simulink model "sedemo_fifo_architectural"  (Simulink 7.5)
settings: Solver=VariableStepDiscrete  StartTime=0.0  StopTime=10  MaxStep=inf  RelTol=1e-3
undefined symbols (not defined in the file or in its folder): des_subsystemblock, des_subsysteminport, des_subsystemoutport, des_subsystemsupportblock
libraries: simeventstranslate1 x16, simeventssink1 x5, simulink x2, simeventsgenerators1 x2, simeventsqueue1 x2, simeventsattributes2 x2, simeventsgates1 x2, simeventsserver1 x2, simeventssignalmanage1 x1, simeventsinfo x1, simeventsrouting1 x1
(part 1 of 2)
settings Model: Creator=The MathWorks Inc.  ExtModeAutoUpdateStatusClock=off
settings DataIOCC: SaveOutput=off  SaveTime=off
settings OptimizationCC: InitFltsAndDblsToZero=on  EfficientMapNaN2IntZero=off
settings DebuggingCC: ReadBeforeWriteMsg=DisableAll  WriteAfterWriteMsg=DisableAll  WriteAfterReadMsg=DisableAll  AlgebraicLoopMsg=error  SolverPrmCheckMsg=none  StrictBusMsg=Warning
settings SimEventsCC: propDiagAttribOutput=1  propDiagFcnCallOutput=1  propDiagStatOutput=0

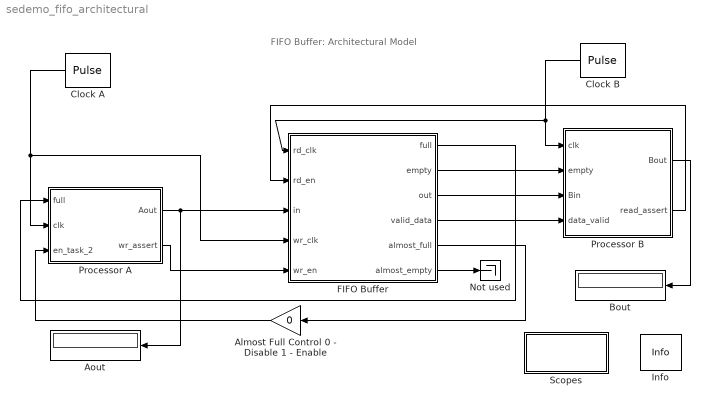
== system sedemo_fifo_architectural ==
  note: FIFO Buffer: Architectural Model
  Almost Full Control 0 - Disable 1 - Enable : Gain  Gain=0  ParameterDataType=sfix(16)  ParameterScaling=2^0  OutDataType=sfix(16)  OutScaling=2^0
  Aout : Display
  Bout : Display
  Clock A : DiscretePulseGenerator  PulseType=Time based  Amplitude=1  Period=0.005  PulseWidth=50  PhaseDelay=0  SampleTime=1
      settings: AttributesFormatString=Period = %<Period>
  Clock B : DiscretePulseGenerator  PulseType=Time based  Amplitude=1  Period=0.0065  PulseWidth=50  PhaseDelay=0  SampleTime=1
      settings: AttributesFormatString=Period = %<Period>
  FIFO Buffer : Subsystem  mask(Variable Capacity, Variable Space per Entity Buffer){thresholdLow=40, thresholdHigh=240, FQcapacity=256}
      mask prompts: thresholdLow "Low Water Level"; thresholdHigh "High Water Level"; FQcapacity "Capacity"
      mask help: Variable capacity queue that allows entities to occupy a variable amount of space per entitiy. The amount of space from an entity is specified from the attribute named in the dialog.
  Info : simeventsinfo/Info  SystemSampleTime=-1
  Not used : Terminator
  Processor A : Subsystem
  Processor B : Subsystem
  Scopes : Subsystem
      settings: RequestExecContextInheritance=on
      mask Display: disp('Scopes');
  wires:
  Clock A/1 -> Processor A/2(clk), FIFO Buffer/4(wr_clk)
  Clock B/1 -> FIFO Buffer/1(rd_clk), Processor B/1(clk)
  FIFO Buffer/3(out) -> Processor B/3(Bin)
  Processor A/1(Aout) -> Aout/1, FIFO Buffer/3(in)
  Processor B/1(Bout) -> Bout/1
  Processor B/2(read_assert) -> FIFO Buffer/2(rd_en)
  Processor A/2(wr_assert) -> FIFO Buffer/5(wr_en)
  FIFO Buffer/1(full) -> Processor A/1(full)
  FIFO Buffer/2(empty) -> Processor B/2(empty)
  FIFO Buffer/4(valid_data) -> Processor B/4(data_valid)
  FIFO Buffer/5(almost_full) -> Almost Full Control 0 - Disable 1 - Enable/1
  FIFO Buffer/6(almost_empty) -> Not used/1
  Almost Full Control 0 - Disable 1 - Enable/1 -> Processor A/3(en_task_2)

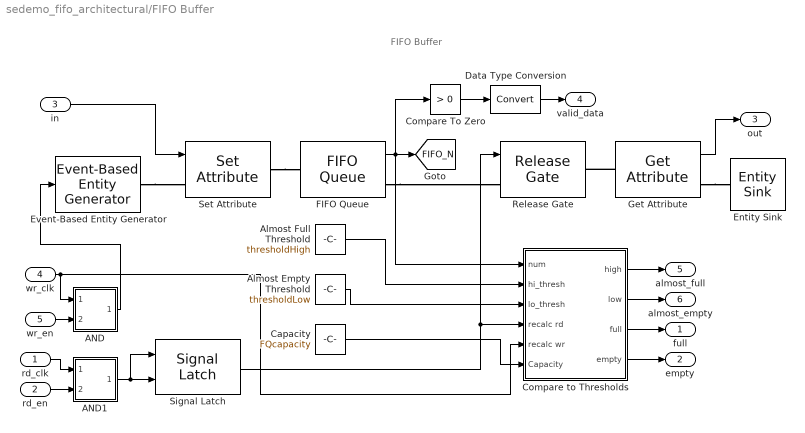
== system sedemo_fifo_architectural/FIFO Buffer ==
  note: FIFO Buffer
  rd_clk : Inport
  rd_en : Inport  Port=2
  in : Inport  Port=3
  wr_clk : Inport  Port=4
  wr_en : Inport  Port=5
  AND : Subsystem  LoadFcn=des_subsystemblock(gcb, 'load');  InitFcn=des_subsystemblock(gcb, 'init');  StartFcn=des_subsystemblock(gcb, 'start');  StopFcn=des_subsystemblock(gcb, 'stop');
      settings: CopyFcn=des_subsystemblock(gcb, 'copy');  DeleteFcn=des_subsystemblock(gcb, 'delete');  UndoDeleteFcn=des_subsystemblock(gcb, 'undodelete');  ModelCloseFcn=des_subsystemblock(gcb, 'modelclose');  PreSaveFcn=des_subsystemblock(gcb, 'presave');  NameChangeFcn=des_subsystemblock(gcb, 'namechange');  OpenFcn=des_subsystemblock(gcb, 'open');  ParentCloseFcn=des_subsystemblock(gcb, 'parentclose');  ErrorFcn=des_subsystemerror
      mask Type: Discrete Event Subsystem
      mask Help: helpview(simeventsbhelp);
  AND1 : Subsystem  LoadFcn=des_subsystemblock(gcb, 'load');  InitFcn=des_subsystemblock(gcb, 'init');  StartFcn=des_subsystemblock(gcb, 'start');  StopFcn=des_subsystemblock(gcb, 'stop');
      settings: CopyFcn=des_subsystemblock(gcb, 'copy');  DeleteFcn=des_subsystemblock(gcb, 'delete');  UndoDeleteFcn=des_subsystemblock(gcb, 'undodelete');  ModelCloseFcn=des_subsystemblock(gcb, 'modelclose');  PreSaveFcn=des_subsystemblock(gcb, 'presave');  NameChangeFcn=des_subsystemblock(gcb, 'namechange');  OpenFcn=des_subsystemblock(gcb, 'open');  ParentCloseFcn=des_subsystemblock(gcb, 'parentclose');  ErrorFcn=des_subsystemerror
      mask Type: Discrete Event Subsystem
      mask Help: helpview(simeventsbhelp);
  Almost Empty Threshold : Constant  Value=thresholdLow  OutDataType=sfix(16)  OutScaling=2^0
  Almost Full Threshold : Constant  Value=thresholdHigh  OutDataType=sfix(16)  OutScaling=2^0
  Capacity : Constant  Value=FQcapacity  OutDataType=sfix(16)  OutScaling=2^0
  Compare To Zero : simulink/Logic and Bit Operations/Compare To Zero  SystemSampleTime=-1  relop=>  LogicOutDataTypeMode=uint8  ZeroCross=off
  Compare to Thresholds : Subsystem  LoadFcn=des_subsystemblock(gcb, 'load');  InitFcn=des_subsystemblock(gcb, 'init');  StartFcn=des_subsystemblock(gcb, 'start');  StopFcn=des_subsystemblock(gcb, 'stop');
      settings: CopyFcn=des_subsystemblock(gcb, 'copy');  DeleteFcn=des_subsystemblock(gcb, 'delete');  UndoDeleteFcn=des_subsystemblock(gcb, 'undodelete');  ModelCloseFcn=des_subsystemblock(gcb, 'modelclose');  PreSaveFcn=des_subsystemblock(gcb, 'presave');  NameChangeFcn=des_subsystemblock(gcb, 'namechange');  OpenFcn=des_subsystemblock(gcb, 'open');  ParentCloseFcn=des_subsystemblock(gcb, 'parentclose');  ErrorFcn=des_subsystemerror
      mask Type: Discrete Event Subsystem
      mask Help: helpview(simeventsbhelp);
  Data Type Conversion : DataTypeConversion  OutDataType=sfix(16)  OutScaling=2^0
  Entity Sink : simeventssink1/Entity Sink  Priority=1  SystemSampleTime=-1  AvailableForArrivals=on  StatNumberArrived=Off
  Event-Based Entity Generator : simeventsgenerators1/Entity Generators/Event-Based Entity Generator  Priority=1  DialogController=des_ddg_create  DialogControllerArgs=DataTag40  SystemSampleTime=-1  GenerateEntitiesUpon=Trigger from port tr  SignalEdgeType=Rising  SpecifyEventPriority=off  PriorityEntityGeneration=300  GenerateEntityAtSimulationStart=off  AllowBlocking=off  ResponseDuringBlockage=Delay first pending entity  EntityType=Blank  StatNumberDeparted=Off  StatPendingEntity=Off  StatAverageIntergenerationTime=Off
  FIFO Queue : simeventsqueue1/FIFO Queue  Priority=1  SystemSampleTime=-1  Capacity=inf  EnableTOPort=off  StatNumberDeparted=Off  StatNumberInBlock=On  StatPendingEntity=Off  StatAverageWait=Off  StatAverageQueueLength=Off  StatNumberTimedout=Off
  Get Attribute : simeventsattributes2/Get Attribute  Priority=1  DialogController=des_ddg_create  DialogControllerArgs=DataTag43  SystemSampleTime=-1  AttributeName=Attribute1  AttributeMissing=Error  AttributeDefaultValue=1  AttributeSendTiming=After entity departure  AttributeTreatAsVector=1  StatNumberDeparted=Off  EvaluatedDefaultAttributeValue={[]}
  Release Gate : simeventsgates1/Release Gate  Priority=1  SystemSampleTime=-1  OpenGateUpon=Trigger from port tr  SignalEdgeOption=Rising  SpecifyEventPriority=off  PriorityGateRelease=2200  StatNumberDeparted=Off
  Set Attribute : simeventsattributes2/Set Attribute  Priority=1  DialogController=des_ddg_create  DialogControllerArgs=DataTag46  SystemSampleTime=-1  AttributeFrom=Signal port|Dialog  AttributeName=Attribute1|space  AttributeTreatAsVector=1|1  AttributeValue=1|1  AttributeCreate=on  StatNumberDeparted=Off  EvaluatedAttributeValue={[];1}
  Signal Latch : simeventssignalmanage1/Signal Latch  SystemSampleTime=-1  InitialMemoryValue=0  WriteMemoryUpon=Sample time hit from port wts  MemoryWriteEdgeOption=Rising  SpecifyWriteEventPriority=on  PriorityMemoryWrite=7100  ReadMemoryUpon=Write to memory event  MemoryReadEdgeOption=Falling  SpecifyReadEventPriority=on  PriorityMemoryRead=7000  ReportMemoryState=off  ReportMemoryUponWrite=off  ReportMemoryUponRead=on
  full : Outport  OutDataType=sfix(16)  OutScaling=2^0
  empty : Outport  Port=2  OutDataType=sfix(16)  OutScaling=2^0
  out : Outport  Port=3
  valid_data : Outport  Port=4  OutDataType=sfix(16)  OutScaling=2^0
  almost_full : Outport  Port=5  OutDataType=sfix(16)  OutScaling=2^0
  almost_empty : Outport  Port=6  OutDataType=sfix(16)  OutScaling=2^0
  tag scope: FIFO_N=global
  wires:
  Almost Full Threshold/1 -> Compare to Thresholds/2(hi_thresh)
  FIFO Queue/1 -> Compare to Thresholds/1(num), [FIFO_N], Compare To Zero/1
  Compare To Zero/1 -> Data Type Conversion/1
  Data Type Conversion/1 -> valid_data/1
  Almost Empty Threshold/1 -> Compare to Thresholds/3(lo_thresh)
  wr_clk/1 -> Compare to Thresholds/5(recalc wr), AND/1(Din)
  Signal Latch/1 -> Compare to Thresholds/4(recalc rd), Release Gate/1
  rd_clk/1 -> AND1/1(Din)
  rd_en/1 -> AND1/2(Din1)
  AND1/1(Dout) -> Signal Latch/2, Signal Latch/1
  wr_en/1 -> AND/2(Din1)
  in/1 -> Set Attribute/1
  Get Attribute/1 -> out/1
  AND/1(Dout) -> Event-Based Entity Generator/1
  Capacity/1 -> Compare to Thresholds/6(Capacity)
  Compare to Thresholds/1(high) -> almost_full/1
  Compare to Thresholds/2(low) -> almost_empty/1
  Compare to Thresholds/3(full) -> full/1
  Compare to Thresholds/4(empty) -> empty/1
  connections:
  Set Attribute/RConn1 -- FIFO Queue/LConn1
  Get Attribute/LConn1 -- Release Gate/RConn1
  FIFO Queue/RConn1 -- Release Gate/LConn1
  Event-Based Entity Generator/RConn1 -- Set Attribute/LConn1
  Get Attribute/RConn1 -- Entity Sink/LConn1

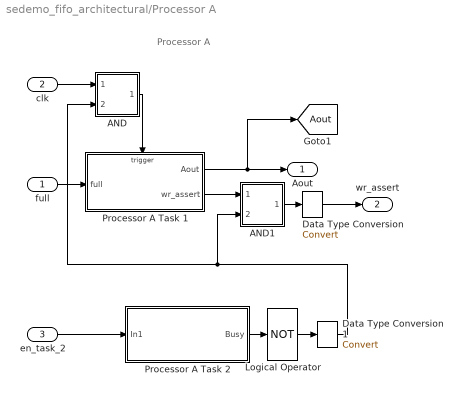
== system sedemo_fifo_architectural/Processor A ==
  note: Processor A
  full : Inport
  clk : Inport  Port=2
  en_task_2 : Inport  Port=3
  AND : Subsystem  LoadFcn=des_subsystemblock(gcb, 'load');  InitFcn=des_subsystemblock(gcb, 'init');  StartFcn=des_subsystemblock(gcb, 'start');  StopFcn=des_subsystemblock(gcb, 'stop');
      settings: CopyFcn=des_subsystemblock(gcb, 'copy');  DeleteFcn=des_subsystemblock(gcb, 'delete');  UndoDeleteFcn=des_subsystemblock(gcb, 'undodelete');  ModelCloseFcn=des_subsystemblock(gcb, 'modelclose');  PreSaveFcn=des_subsystemblock(gcb, 'presave');  NameChangeFcn=des_subsystemblock(gcb, 'namechange');  OpenFcn=des_subsystemblock(gcb, 'open');  ParentCloseFcn=des_subsystemblock(gcb, 'parentclose');  ErrorFcn=des_subsystemerror
      mask Type: Discrete Event Subsystem
      mask Help: helpview(simeventsbhelp);
  AND1 : Subsystem  LoadFcn=des_subsystemblock(gcb, 'load');  InitFcn=des_subsystemblock(gcb, 'init');  StartFcn=des_subsystemblock(gcb, 'start');  StopFcn=des_subsystemblock(gcb, 'stop');
      settings: CopyFcn=des_subsystemblock(gcb, 'copy');  DeleteFcn=des_subsystemblock(gcb, 'delete');  UndoDeleteFcn=des_subsystemblock(gcb, 'undodelete');  ModelCloseFcn=des_subsystemblock(gcb, 'modelclose');  PreSaveFcn=des_subsystemblock(gcb, 'presave');  NameChangeFcn=des_subsystemblock(gcb, 'namechange');  OpenFcn=des_subsystemblock(gcb, 'open');  ParentCloseFcn=des_subsystemblock(gcb, 'parentclose');  ErrorFcn=des_subsystemerror
      mask Type: Discrete Event Subsystem
      mask Help: helpview(simeventsbhelp);
  Data Type Conversion : DataTypeConversion  OutDataType=sfix(16)  OutScaling=2^0
  Data Type Conversion1 : DataTypeConversion  OutDataType=sfix(16)  OutScaling=2^0
  Logical Operator : Logic  Operator=NOT  AllPortsSameDT=off  OutDataTypeMode=boolean  OutDataTypeStr=boolean
  Processor A Task 1 : Subsystem  TreatAsAtomicUnit=on
      settings: PropExecContextOutsideSubsystem=on
  Processor A Task 2 : Subsystem
  Aout : Outport
  wr_assert : Outport  Port=2
  tag scope: Aout=global
  wires:
  Processor A Task 1/1(Aout) -> Aout/1, [Aout]
  full/1 -> Processor A Task 1/1(full)
  en_task_2/1 -> Processor A Task 2/1(In1)
  Processor A Task 2/1(Busy) -> Logical Operator/1
  AND/1(Dout) -> Processor A Task 1/Trigger
  clk/1 -> AND/1(Din)
  AND1/1(Dout) -> Data Type Conversion/1
  Processor A Task 1/2(wr_assert) -> AND1/1(Din)
  Data Type Conversion/1 -> wr_assert/1
  Logical Operator/1 -> Data Type Conversion1/1
  Data Type Conversion1/1 -> AND/2(Din1), AND1/2(Din1)

== system sedemo_fifo_architectural/Processor B ==
  note: Processor B
  clk : Inport
  empty : Inport  Port=2
  Bin : Inport  Port=3
  data_valid : Inport  Port=4
  Not used : Terminator
  Processor B Task : Subsystem  TreatAsAtomicUnit=on
      settings: PropExecContextOutsideSubsystem=on
  Bout : Outport
  read_assert : Outport  Port=2
  tag scope: Bout=global
  wires:
  Bin/1 -> Processor B Task/1(Bin)
  Processor B Task/1(Cout) -> Bout/1, [Bout]
  data_valid/1 -> Not used/1
  empty/1 -> Processor B Task/2(empty)
  Processor B Task/2(read_assert) -> read_assert/1
  clk/1 -> Processor B Task/Trigger

== system sedemo_fifo_architectural/Scopes ==
  Buffer Size : simeventssink1/Signal Scope  Priority=1  SystemSampleTime=-1  PlotType=Stair  InputType=Signal  NumInputs=1  AttributeNameY=Count  XInputOptionSignal=Event time  XInputOptionEntity=Event time  AttributeNameX=Count  EnableEntityOutport=on  XMin=-0.0999478213651573  XMax=10.0947299578809  XLimitExceededOption=Stretch axis limits  YLimitExceededOption=Stretch axis limits  AxisGrid=on  AxisLegend=off  LineDisables=""  LineColors=b  LineStyles=-  LineMarkers=.  OpenScopeAtSimStart=on  Title=Number in Buffer  YLabel=#n  XLabel=Time  FigurePosition=[51 228 231 131]  AxisZoom=off  DataStoreOption=Limited  DataPointsLimit=10000  StatNumberArrived=Off  ShowCountPlotted=off  ShowToolbar=off
      settings: YMin=-2.05  YMax=3.05
  Discrete Event Subsystem Difference : Subsystem  LoadFcn=des_subsystemblock(gcb, 'load');  InitFcn=des_subsystemblock(gcb, 'init');  StartFcn=des_subsystemblock(gcb, 'start');  StopFcn=des_subsystemblock(gcb, 'stop');
      settings: CopyFcn=des_subsystemblock(gcb, 'copy');  DeleteFcn=des_subsystemblock(gcb, 'delete');  UndoDeleteFcn=des_subsystemblock(gcb, 'undodelete');  ModelCloseFcn=des_subsystemblock(gcb, 'modelclose');  PreSaveFcn=des_subsystemblock(gcb, 'presave');  NameChangeFcn=des_subsystemblock(gcb, 'namechange');  OpenFcn=des_subsystemblock(gcb, 'open');  ParentCloseFcn=des_subsystemblock(gcb, 'parentclose');  ErrorFcn=des_subsystemerror
      mask Type: Discrete Event Subsystem
      mask Help: helpview(simeventsbhelp);
  Value of 'A' : simeventssink1/Signal Scope  Priority=1  SystemSampleTime=-1  PlotType=Stair  InputType=Signal  NumInputs=1  AttributeNameY=Count  XInputOptionSignal=Event time  XInputOptionEntity=Event time  AttributeNameX=Count  EnableEntityOutport=on  XMin=-0.0999478213651573  XMax=10.0947299578809  XLimitExceededOption=Stretch axis limits  YLimitExceededOption=Stretch axis limits  AxisGrid=on  AxisLegend=off  LineDisables=""  LineColors=b  LineStyles=-  LineMarkers=.  OpenScopeAtSimStart=on  Title=Value of 'A'  YLabel=""  XLabel=Time  FigurePosition=[294 227 232 134]  AxisZoom=off  DataStoreOption=Limited  DataPointsLimit=10000  StatNumberArrived=Off  ShowCountPlotted=off  ShowToolbar=off
      settings: YMin=-2.05  YMax=3.05
  Value of 'A' - 'B' : simeventssink1/Signal Scope  Priority=1  SystemSampleTime=-1  PlotType=Stair  InputType=Signal  NumInputs=1  AttributeNameY=Count  XInputOptionSignal=Event time  XInputOptionEntity=Event time  AttributeNameX=Count  EnableEntityOutport=on  XMin=-0.0999478213651573  XMax=10.0947299578809  XLimitExceededOption=Stretch axis limits  YLimitExceededOption=Stretch axis limits  AxisGrid=on  AxisLegend=off  LineDisables=""  LineColors=b  LineStyles=-  LineMarkers=.  OpenScopeAtSimStart=on  Title=Value of 'A' - 'B'  YLabel='A' - 'B'  XLabel=Time  FigurePosition=[50 65 231 135]  AxisZoom=off  DataStoreOption=Limited  DataPointsLimit=10000  StatNumberArrived=Off  ShowCountPlotted=off  ShowToolbar=off
      settings: YMin=-2.05  YMax=3.05
  Value of 'B' : simeventssink1/Signal Scope  Priority=1  SystemSampleTime=-1  PlotType=Stair  InputType=Signal  NumInputs=1  AttributeNameY=Count  XInputOptionSignal=Event time  XInputOptionEntity=Event time  AttributeNameX=Count  EnableEntityOutport=on  XMin=-0.0999478213651573  XMax=10.0947299578809  XLimitExceededOption=Stretch axis limits  YLimitExceededOption=Stretch axis limits  AxisGrid=on  AxisLegend=off  LineDisables=""  LineColors=b  LineStyles=-  LineMarkers=.  OpenScopeAtSimStart=on  Title=Value of 'B'  YLabel=""  XLabel=Time  FigurePosition=[294 66 230 136]  AxisZoom=off  DataStoreOption=Limited  DataPointsLimit=10000  StatNumberArrived=Off  ShowCountPlotted=off  ShowToolbar=off
      settings: YMin=-2.05  YMax=3.05
  wires:
  Discrete Event Subsystem Difference/1(Dout) -> Value of 'A' - 'B'/1
  [Aout] -> Discrete Event Subsystem Difference/1(Din), Value of 'A'/1
  [Bout] -> Discrete Event Subsystem Difference/2(Din1), Value of 'B'/1
  [FIFO_N] -> Buffer Size/1

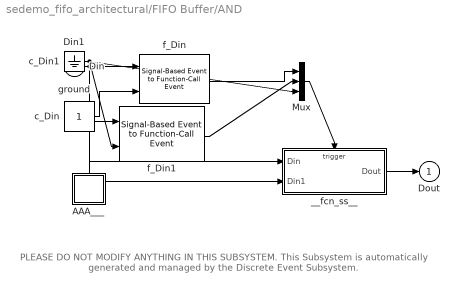
== system sedemo_fifo_architectural/FIFO Buffer/AND ==
  note: PLEASE DO NOT MODIFY ANYTHING IN THIS SUBSYSTEM.
      | This Subsystem is automatically generated and
      | managed by the Discrete Event Subsystem.
  Din : Inport  DataType=double  OutDataType=sfix(16)  OutScaling=2^0  OutDataTypeStr=double
  Din1 : Inport  Port=2  DataType=double  OutDataTypeStr=double
  AAA___ : Subsystem  LoadFcn=des_subsystemsupportblock(gcb, 'load');  InitFcn=des_subsystemsupportblock(gcb, 'init');  StartFcn=des_subsystemsupportblock(gcb, 'start');  StopFcn=des_subsystemsupportblock(gcb, 'stop');
      settings: CopyFcn=des_subsystemsupportblock(gcb, 'copy');  DeleteFcn=des_subsystemsupportblock(gcb, 'delete');  UndoDeleteFcn=des_subsystemsupportblock(gcb, 'undodelete');  ModelCloseFcn=des_subsystemsupportblock(gcb, 'modelclose');  PreSaveFcn=des_subsystemsupportblock(gcb, 'presave');  NameChangeFcn=des_subsystemsupportblock(gcb, 'namechange');  OpenFcn=des_subsystemsupportblock(gcb, 'open');  ParentCloseFcn=des_subsystemsupportblock(gcb, 'parentclose');
  Mux : Mux  Inputs=3
  __fcn_ss__ : Subsystem  TreatAsAtomicUnit=on
      settings: PropExecContextOutsideSubsystem=on
  c_Din : Constant  OutDataType=sfix(16)  OutScaling=2^0
  c_Din1 : Constant
  f_Din : simeventstranslate1/Signal-Based Event to Function-Call Event  Priority=1  SystemSampleTime=-1  GenerateFunctionCallUpon=Sample time hit from port ts  SignalEdgeOption=Rising  EnableE1Port=on  EnableF2Port=off  EnableE2Port=off  SpecifyEventPriority=off  PriorityFunctionCall=20  FunctionCallDelayFrom=Dialog  DelayFunctionCall=0  StatNumberF1Calls=Off  StatNumberF2Calls=Off  MaskBlockType=DESS_EVENT_PORT
  f_Din1 : simeventstranslate1/Signal-Based Event to Function-Call Event  Priority=1  SystemSampleTime=-1  GenerateFunctionCallUpon=Sample time hit from port ts  SignalEdgeOption=Rising  EnableE1Port=on  EnableF2Port=off  EnableE2Port=off  SpecifyEventPriority=off  PriorityFunctionCall=20  FunctionCallDelayFrom=Dialog  DelayFunctionCall=0  StatNumberF1Calls=Off  StatNumberF2Calls=Off  MaskBlockType=DESS_EVENT_PORT
  ground : Ground
  Dout : Outport  OutDataType=sfix(16)  OutScaling=2^0
  wires:
  __fcn_ss__/1(Dout) -> Dout/1
  f_Din/1 -> Mux/1
  c_Din/1 -> f_Din/2
  Mux/1 -> __fcn_ss__/Trigger
  f_Din1/1 -> Mux/2
  c_Din1/1 -> f_Din1/2
  ground/1 -> Mux/3
  Din/1 -> f_Din/1, __fcn_ss__/1(Din)
  Din1/1 -> f_Din1/1, __fcn_ss__/2(Din1)

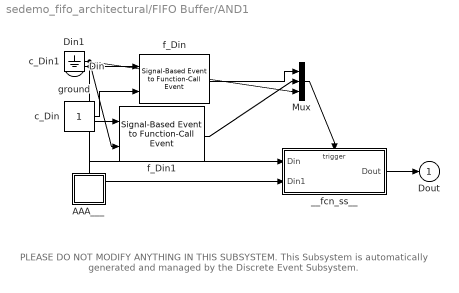
== system sedemo_fifo_architectural/FIFO Buffer/AND1 ==
  note: PLEASE DO NOT MODIFY ANYTHING IN THIS SUBSYSTEM.
      | This Subsystem is automatically generated and
      | managed by the Discrete Event Subsystem.
  Din : Inport  DataType=double  OutDataType=sfix(16)  OutScaling=2^0  OutDataTypeStr=double
  Din1 : Inport  Port=2  DataType=double  OutDataTypeStr=double
  AAA___ : Subsystem  LoadFcn=des_subsystemsupportblock(gcb, 'load');  InitFcn=des_subsystemsupportblock(gcb, 'init');  StartFcn=des_subsystemsupportblock(gcb, 'start');  StopFcn=des_subsystemsupportblock(gcb, 'stop');
      settings: CopyFcn=des_subsystemsupportblock(gcb, 'copy');  DeleteFcn=des_subsystemsupportblock(gcb, 'delete');  UndoDeleteFcn=des_subsystemsupportblock(gcb, 'undodelete');  ModelCloseFcn=des_subsystemsupportblock(gcb, 'modelclose');  PreSaveFcn=des_subsystemsupportblock(gcb, 'presave');  NameChangeFcn=des_subsystemsupportblock(gcb, 'namechange');  OpenFcn=des_subsystemsupportblock(gcb, 'open');  ParentCloseFcn=des_subsystemsupportblock(gcb, 'parentclose');
  Mux : Mux  Inputs=3
  __fcn_ss__ : Subsystem  TreatAsAtomicUnit=on
      settings: PropExecContextOutsideSubsystem=on
  c_Din : Constant  OutDataType=sfix(16)  OutScaling=2^0
  c_Din1 : Constant
  f_Din : simeventstranslate1/Signal-Based Event to Function-Call Event  Priority=1  SystemSampleTime=-1  GenerateFunctionCallUpon=Sample time hit from port ts  SignalEdgeOption=Rising  EnableE1Port=on  EnableF2Port=off  EnableE2Port=off  SpecifyEventPriority=off  PriorityFunctionCall=20  FunctionCallDelayFrom=Dialog  DelayFunctionCall=0  StatNumberF1Calls=Off  StatNumberF2Calls=Off  MaskBlockType=DESS_EVENT_PORT
  f_Din1 : simeventstranslate1/Signal-Based Event to Function-Call Event  Priority=1  SystemSampleTime=-1  GenerateFunctionCallUpon=Sample time hit from port ts  SignalEdgeOption=Rising  EnableE1Port=on  EnableF2Port=off  EnableE2Port=off  SpecifyEventPriority=off  PriorityFunctionCall=20  FunctionCallDelayFrom=Dialog  DelayFunctionCall=0  StatNumberF1Calls=Off  StatNumberF2Calls=Off  MaskBlockType=DESS_EVENT_PORT
  ground : Ground
  Dout : Outport  OutDataType=sfix(16)  OutScaling=2^0
  wires:
  __fcn_ss__/1(Dout) -> Dout/1
  f_Din/1 -> Mux/1
  c_Din/1 -> f_Din/2
  Mux/1 -> __fcn_ss__/Trigger
  f_Din1/1 -> Mux/2
  c_Din1/1 -> f_Din1/2
  ground/1 -> Mux/3
  Din/1 -> f_Din/1, __fcn_ss__/1(Din)
  Din1/1 -> f_Din1/1, __fcn_ss__/2(Din1)

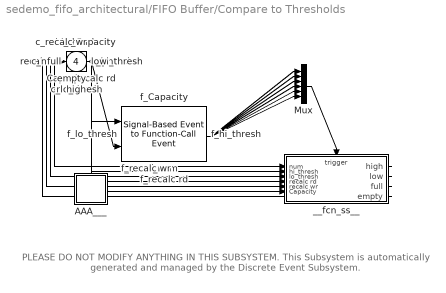
== system sedemo_fifo_architectural/FIFO Buffer/Compare to Thresholds ==
  note: PLEASE DO NOT MODIFY ANYTHING IN THIS SUBSYSTEM.
      | This Subsystem is automatically generated and
      | managed by the Discrete Event Subsystem.
  num : Inport  DataType=double  OutDataTypeStr=double
  hi_thresh : Inport  Port=2  DataType=double  OutDataTypeStr=double
  lo_thresh : Inport  Port=3  DataType=double  OutDataTypeStr=double
  recalc rd : Inport  Port=4  DataType=double  OutDataTypeStr=double
  recalc wr : Inport  Port=5  DataType=double  OutDataTypeStr=double
  Capacity : Inport  Port=6  DataType=double  OutDataTypeStr=double
  AAA___ : Subsystem  LoadFcn=des_subsystemsupportblock(gcb, 'load');  InitFcn=des_subsystemsupportblock(gcb, 'init');  StartFcn=des_subsystemsupportblock(gcb, 'start');  StopFcn=des_subsystemsupportblock(gcb, 'stop');
      settings: CopyFcn=des_subsystemsupportblock(gcb, 'copy');  DeleteFcn=des_subsystemsupportblock(gcb, 'delete');  UndoDeleteFcn=des_subsystemsupportblock(gcb, 'undodelete');  ModelCloseFcn=des_subsystemsupportblock(gcb, 'modelclose');  PreSaveFcn=des_subsystemsupportblock(gcb, 'presave');  NameChangeFcn=des_subsystemsupportblock(gcb, 'namechange');  OpenFcn=des_subsystemsupportblock(gcb, 'open');  ParentCloseFcn=des_subsystemsupportblock(gcb, 'parentclose');
  Mux : Mux  Inputs=6
  __fcn_ss__ : Subsystem  TreatAsAtomicUnit=on
      settings: PropExecContextOutsideSubsystem=on
  c_Capacity : Constant  Value=0
  c_hi_thresh : Constant  Value=0
  c_lo_thresh : Constant  Value=0
  c_num : Constant
  c_recalc rd : Constant
  c_recalc wr : Constant
  f_Capacity : simeventstranslate1/Signal-Based Event to Function-Call Event  Priority=1  SystemSampleTime=-1  GenerateFunctionCallUpon=Sample time hit from port ts  SignalEdgeOption=Rising  EnableE1Port=on  EnableF2Port=off  EnableE2Port=off  SpecifyEventPriority=off  PriorityFunctionCall=200  FunctionCallDelayFrom=Dialog  DelayFunctionCall=0  StatNumberF1Calls=Off  StatNumberF2Calls=Off  MaskBlockType=DESS_DATA_PORT
  f_hi_thresh : simeventstranslate1/Signal-Based Event to Function-Call Event  Priority=1  SystemSampleTime=-1  GenerateFunctionCallUpon=Sample time hit from port ts  SignalEdgeOption=Rising  EnableE1Port=on  EnableF2Port=off  EnableE2Port=off  SpecifyEventPriority=off  PriorityFunctionCall=20  FunctionCallDelayFrom=Dialog  DelayFunctionCall=0  StatNumberF1Calls=Off  StatNumberF2Calls=Off  MaskBlockType=DESS_DATA_PORT
  f_lo_thresh : simeventstranslate1/Signal-Based Event to Function-Call Event  Priority=1  SystemSampleTime=-1  GenerateFunctionCallUpon=Sample time hit from port ts  SignalEdgeOption=Rising  EnableE1Port=on  EnableF2Port=off  EnableE2Port=off  SpecifyEventPriority=off  PriorityFunctionCall=20  FunctionCallDelayFrom=Dialog  DelayFunctionCall=0  StatNumberF1Calls=Off  StatNumberF2Calls=Off  MaskBlockType=DESS_DATA_PORT
  f_num : simeventstranslate1/Signal-Based Event to Function-Call Event  Priority=1  SystemSampleTime=-1  GenerateFunctionCallUpon=Sample time hit from port ts  SignalEdgeOption=Rising  EnableE1Port=on  EnableF2Port=off  EnableE2Port=off  SpecifyEventPriority=off  PriorityFunctionCall=20  FunctionCallDelayFrom=Dialog  DelayFunctionCall=0  StatNumberF1Calls=Off  StatNumberF2Calls=Off  MaskBlockType=DESS_EVENT_PORT
  f_recalc rd : simeventstranslate1/Signal-Based Event to Function-Call Event  Priority=1  SystemSampleTime=-1  GenerateFunctionCallUpon=Trigger from port tr  SignalEdgeOption=Rising  EnableE1Port=on  EnableF2Port=off  EnableE2Port=off  SpecifyEventPriority=off  PriorityFunctionCall=20  FunctionCallDelayFrom=Dialog  DelayFunctionCall=0  StatNumberF1Calls=Off  StatNumberF2Calls=Off  MaskBlockType=DESS_EVENT_PORT
  f_recalc wr : simeventstranslate1/Signal-Based Event to Function-Call Event  Priority=1  SystemSampleTime=-1  GenerateFunctionCallUpon=Trigger from port tr  SignalEdgeOption=Rising  EnableE1Port=on  EnableF2Port=off  EnableE2Port=off  SpecifyEventPriority=off  PriorityFunctionCall=20  FunctionCallDelayFrom=Dialog  DelayFunctionCall=0  StatNumberF1Calls=Off  StatNumberF2Calls=Off  MaskBlockType=DESS_EVENT_PORT
  high : Outport
  low : Outport  Port=2
  full : Outport  Port=3
  empty : Outport  Port=4
  wires:
  Mux/1 -> __fcn_ss__/Trigger
  f_num/1 -> Mux/2
  c_num/1 -> f_num/2
  __fcn_ss__/1(high) -> high/1
  f_hi_thresh/1 -> Mux/3
  c_hi_thresh/1 -> f_hi_thresh/2
  hi_thresh/1 -> f_hi_thresh/1, __fcn_ss__/2(hi_thresh)
  __fcn_ss__/2(low) -> low/1
  f_lo_thresh/1 -> Mux/4
  c_lo_thresh/1 -> f_lo_thresh/2
  lo_thresh/1 -> f_lo_thresh/1, __fcn_ss__/3(lo_thresh)
  f_recalc rd/1 -> Mux/5
  c_recalc rd/1 -> f_recalc rd/2
  f_recalc wr/1 -> Mux/6
  c_recalc wr/1 -> f_recalc wr/2
  Capacity/1 -> f_Capacity/1, __fcn_ss__/6(Capacity)
  f_Capacity/1 -> Mux/1
  c_Capacity/1 -> f_Capacity/2
  __fcn_ss__/3(full) -> full/1
  __fcn_ss__/4(empty) -> empty/1
  num/1 -> f_num/1, __fcn_ss__/1(num)
  recalc rd/1 -> f_recalc rd/1, __fcn_ss__/4(recalc rd)
  recalc wr/1 -> f_recalc wr/1, __fcn_ss__/5(recalc wr)

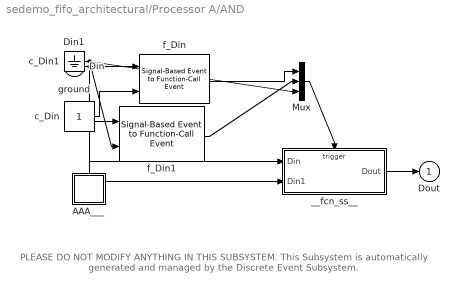
== system sedemo_fifo_architectural/Processor A/AND ==
  note: PLEASE DO NOT MODIFY ANYTHING IN THIS SUBSYSTEM.
      | This Subsystem is automatically generated and
      | managed by the Discrete Event Subsystem.
  Din : Inport  DataType=double  OutDataType=sfix(16)  OutScaling=2^0  OutDataTypeStr=double
  Din1 : Inport  Port=2  DataType=double  OutDataTypeStr=double
  AAA___ : Subsystem  LoadFcn=des_subsystemsupportblock(gcb, 'load');  InitFcn=des_subsystemsupportblock(gcb, 'init');  StartFcn=des_subsystemsupportblock(gcb, 'start');  StopFcn=des_subsystemsupportblock(gcb, 'stop');
      settings: CopyFcn=des_subsystemsupportblock(gcb, 'copy');  DeleteFcn=des_subsystemsupportblock(gcb, 'delete');  UndoDeleteFcn=des_subsystemsupportblock(gcb, 'undodelete');  ModelCloseFcn=des_subsystemsupportblock(gcb, 'modelclose');  PreSaveFcn=des_subsystemsupportblock(gcb, 'presave');  NameChangeFcn=des_subsystemsupportblock(gcb, 'namechange');  OpenFcn=des_subsystemsupportblock(gcb, 'open');  ParentCloseFcn=des_subsystemsupportblock(gcb, 'parentclose');
  Mux : Mux  Inputs=3
  __fcn_ss__ : Subsystem  TreatAsAtomicUnit=on
      settings: PropExecContextOutsideSubsystem=on
  c_Din : Constant  OutDataType=sfix(16)  OutScaling=2^0
  c_Din1 : Constant
  f_Din : simeventstranslate1/Signal-Based Event to Function-Call Event  Priority=1  SystemSampleTime=-1  GenerateFunctionCallUpon=Sample time hit from port ts  SignalEdgeOption=Rising  EnableE1Port=on  EnableF2Port=off  EnableE2Port=off  SpecifyEventPriority=off  PriorityFunctionCall=20  FunctionCallDelayFrom=Dialog  DelayFunctionCall=0  StatNumberF1Calls=Off  StatNumberF2Calls=Off  MaskBlockType=DESS_EVENT_PORT
  f_Din1 : simeventstranslate1/Signal-Based Event to Function-Call Event  Priority=1  SystemSampleTime=-1  GenerateFunctionCallUpon=Sample time hit from port ts  SignalEdgeOption=Rising  EnableE1Port=on  EnableF2Port=off  EnableE2Port=off  SpecifyEventPriority=off  PriorityFunctionCall=20  FunctionCallDelayFrom=Dialog  DelayFunctionCall=0  StatNumberF1Calls=Off  StatNumberF2Calls=Off  MaskBlockType=DESS_EVENT_PORT
  ground : Ground
  Dout : Outport  OutDataType=sfix(16)  OutScaling=2^0
  wires:
  __fcn_ss__/1(Dout) -> Dout/1
  f_Din/1 -> Mux/1
  c_Din/1 -> f_Din/2
  Mux/1 -> __fcn_ss__/Trigger
  f_Din1/1 -> Mux/2
  c_Din1/1 -> f_Din1/2
  ground/1 -> Mux/3
  Din/1 -> f_Din/1, __fcn_ss__/1(Din)
  Din1/1 -> f_Din1/1, __fcn_ss__/2(Din1)

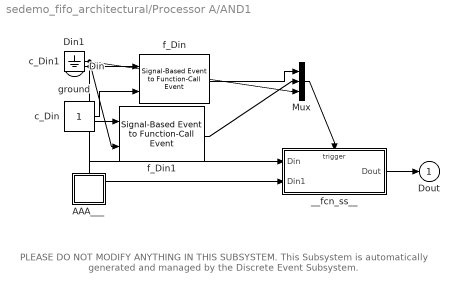
== system sedemo_fifo_architectural/Processor A/AND1 ==
  note: PLEASE DO NOT MODIFY ANYTHING IN THIS SUBSYSTEM.
      | This Subsystem is automatically generated and
      | managed by the Discrete Event Subsystem.
  Din : Inport  DataType=double  OutDataType=sfix(16)  OutScaling=2^0  OutDataTypeStr=double
  Din1 : Inport  Port=2  DataType=double  OutDataTypeStr=double
  AAA___ : Subsystem  LoadFcn=des_subsystemsupportblock(gcb, 'load');  InitFcn=des_subsystemsupportblock(gcb, 'init');  StartFcn=des_subsystemsupportblock(gcb, 'start');  StopFcn=des_subsystemsupportblock(gcb, 'stop');
      settings: CopyFcn=des_subsystemsupportblock(gcb, 'copy');  DeleteFcn=des_subsystemsupportblock(gcb, 'delete');  UndoDeleteFcn=des_subsystemsupportblock(gcb, 'undodelete');  ModelCloseFcn=des_subsystemsupportblock(gcb, 'modelclose');  PreSaveFcn=des_subsystemsupportblock(gcb, 'presave');  NameChangeFcn=des_subsystemsupportblock(gcb, 'namechange');  OpenFcn=des_subsystemsupportblock(gcb, 'open');  ParentCloseFcn=des_subsystemsupportblock(gcb, 'parentclose');
  Mux : Mux  Inputs=3
  __fcn_ss__ : Subsystem  TreatAsAtomicUnit=on
      settings: PropExecContextOutsideSubsystem=on
  c_Din : Constant  OutDataType=sfix(16)  OutScaling=2^0
  c_Din1 : Constant
  f_Din : simeventstranslate1/Signal-Based Event to Function-Call Event  Priority=1  SystemSampleTime=-1  GenerateFunctionCallUpon=Sample time hit from port ts  SignalEdgeOption=Rising  EnableE1Port=on  EnableF2Port=off  EnableE2Port=off  SpecifyEventPriority=off  PriorityFunctionCall=20  FunctionCallDelayFrom=Dialog  DelayFunctionCall=0  StatNumberF1Calls=Off  StatNumberF2Calls=Off  MaskBlockType=DESS_EVENT_PORT
  f_Din1 : simeventstranslate1/Signal-Based Event to Function-Call Event  Priority=1  SystemSampleTime=-1  GenerateFunctionCallUpon=Sample time hit from port ts  SignalEdgeOption=Rising  EnableE1Port=on  EnableF2Port=off  EnableE2Port=off  SpecifyEventPriority=off  PriorityFunctionCall=20  FunctionCallDelayFrom=Dialog  DelayFunctionCall=0  StatNumberF1Calls=Off  StatNumberF2Calls=Off  MaskBlockType=DESS_EVENT_PORT
  ground : Ground
  Dout : Outport  OutDataType=sfix(16)  OutScaling=2^0
  wires:
  __fcn_ss__/1(Dout) -> Dout/1
  f_Din/1 -> Mux/1
  c_Din/1 -> f_Din/2
  Mux/1 -> __fcn_ss__/Trigger
  f_Din1/1 -> Mux/2
  c_Din1/1 -> f_Din1/2
  ground/1 -> Mux/3
  Din/1 -> f_Din/1, __fcn_ss__/1(Din)
  Din1/1 -> f_Din1/1, __fcn_ss__/2(Din1)

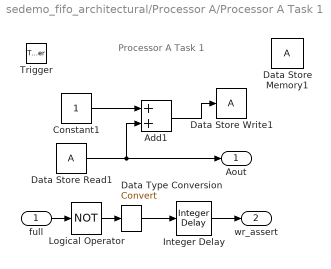
== system sedemo_fifo_architectural/Processor A/Processor A Task 1 ==
  note: Processor A
      | Task 1
  full : Inport
  Trigger : TriggerPort
  Add1 : Sum  OutDataType=sfix(16)  OutScaling=2^-10
  Constant1 : Constant  OutDataType=sfix(16)  OutScaling=2^0
  Data Store Memory1 : DataStoreMemory  DataStoreName=A  ReadBeforeWriteMsg=warning  WriteAfterWriteMsg=warning  WriteAfterReadMsg=warning  OutDataType=sfix(16)  OutScaling=2^0
  Data Store Read1 : DataStoreRead  DataStoreName=A  SampleTime=-1
  Data Store Write1 : DataStoreWrite  DataStoreName=A  SampleTime=-1
  Data Type Conversion : DataTypeConversion  OutDataType=sfix(16)  OutScaling=2^0
  Integer Delay : simulink/Discrete/Integer Delay  vinit=1  samptime=-1  NumDelays=8
  Logical Operator : Logic  Operator=NOT  AllPortsSameDT=off  OutDataTypeMode=boolean  OutDataTypeStr=boolean
  Aout : Outport  OutDataType=sfix(16)  OutScaling=2^0
  wr_assert : Outport  Port=2
  wires:
  Add1/1 -> Data Store Write1/1
  Constant1/1 -> Add1/1
  Data Store Read1/1 -> Aout/1, Add1/2
  full/1 -> Logical Operator/1
  Logical Operator/1 -> Data Type Conversion/1
  Data Type Conversion/1 -> Integer Delay/1
  Integer Delay/1 -> wr_assert/1

== system sedemo_fifo_architectural/Processor A/Processor A Task 2 ==
  note: Processor A Task 2
  In1 : Inport
  Enabled Gate Start Task if '1' : simeventsgates1/Enabled Gate  Priority=1  SystemSampleTime=-1  SpecifyEventPriority=off  PriorityGateEnableOpenClose=2000  StatNumberDeparted=Off
  FIFO Queue : simeventsqueue1/FIFO Queue  Priority=1  SystemSampleTime=-1  Capacity=1  EnableTOPort=off  StatNumberDeparted=Off  StatNumberInBlock=Off  StatPendingEntity=Off  StatAverageWait=Off  StatAverageQueueLength=Off  StatNumberTimedout=Off
  Path Combiner : simeventsrouting1/Path Combiner  Priority=1  SystemSampleTime=-1  NumberInputPorts=2  InputPortPrecedence=IN1 port  InitialSeed=45675  SpecifyEventPriority=off  PriorityPathCombinerPortPrecedenceSelection=4100  StatNumberDeparted=Off  StatLastArrivalPort=Off  EvaluatedNumPorts=2
  Single Server Delay to switch tasks : simeventsserver1/Single Server  Priority=1  SystemSampleTime=-1  ServiceTimeFrom=Dialog  ServiceTime=0.064  AttributeName=ServiceTime  PriorityServiceCompletion=500  PermitPreemption=off  SortingAttributeName=PriorityAttributeName  SortingDirection=Ascending  WriteToAttribute=off  ResidualAttributeName=ResidualServiceTime  CreateAttribute=on  EnableTOPort=off  StatNumberDeparted=Off  StatNumberInBlock=Off  StatNumberPreempted=Off  StatPendingEntity=Off  StatAverageWait=Off  StatUtilization=Off  StatNumberTimedout=Off
      settings: AttributesFormatString=Service Time = %<ServiceTime>
  Single Server Task Time : simeventsserver1/Single Server  Priority=1  SystemSampleTime=-1  ServiceTimeFrom=Dialog  ServiceTime=0.25  AttributeName=ServiceTime  PriorityServiceCompletion=500  PermitPreemption=off  SortingAttributeName=PriorityAttributeName  SortingDirection=Ascending  WriteToAttribute=off  ResidualAttributeName=ResidualServiceTime  CreateAttribute=on  EnableTOPort=off  StatNumberDeparted=Off  StatNumberInBlock=On  StatNumberPreempted=Off  StatPendingEntity=Off  StatAverageWait=Off  StatUtilization=Off  StatNumberTimedout=Off
      settings: AttributesFormatString=Service Time = %<ServiceTime>
  Time-Based Entity Generator : simeventsgenerators1/Entity Generators/Time-Based Entity Generator  Priority=1  DialogController=des_ddg_create  DialogControllerArgs=DataTag72  SystemSampleTime=-1  GenerateEntitiesUpon=Intergeneration time from dialog  Distribution=Constant  Minimum=0  Maximum=1  Mean=1  InitialSeed=12345  Period=inf  PriorityEntityGeneration=300  GenerateEntityAtSimulationStart=on  ResponseWhenBlocked=Pause generation  ResponseWhenUnblocked=Immediate restart  EntityType=Blank  StatNumberDeparted=Off  StatPendingEntity=Off  StatAverageIntergenerationTime=Off
      settings: AttributesFormatString=Period = %<Period>
  Busy : Outport
  wires:
  In1/1 -> Enabled Gate Start Task if '1'/1
  Single Server Task Time/1 -> Busy/1
  connections:
  Path Combiner/LConn1 -- Time-Based Entity Generator/RConn1
  Path Combiner/LConn2 -- Single Server Task Time/RConn1
  FIFO Queue/LConn1 -- Path Combiner/RConn1
  FIFO Queue/RConn1 -- Enabled Gate Start Task if '1'/LConn1
  Single Server Delay to switch tasks/RConn1 -- Single Server Task Time/LConn1
  Enabled Gate Start Task if '1'/RConn1 -- Single Server Delay to switch tasks/LConn1

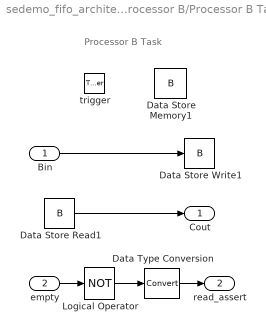
== system sedemo_fifo_architectural/Processor B/Processor B Task ==
  note: Processor B Task
  Bin : Inport
  empty : Inport  Port=2
  trigger : TriggerPort
  Data Store Memory1 : DataStoreMemory  DataStoreName=B  ReadBeforeWriteMsg=warning  WriteAfterWriteMsg=warning  WriteAfterReadMsg=warning  OutDataType=sfix(16)  OutScaling=2^0
  Data Store Read1 : DataStoreRead  DataStoreName=B  SampleTime=-1
  Data Store Write1 : DataStoreWrite  DataStoreName=B  SampleTime=-1
  Data Type Conversion : DataTypeConversion  OutDataType=sfix(16)  OutScaling=2^0
  Logical Operator : Logic  Operator=NOT  AllPortsSameDT=off  OutDataTypeMode=boolean  OutDataTypeStr=boolean
  Cout : Outport  OutDataType=sfix(16)  OutScaling=2^0
  read_assert : Outport  Port=2
  wires:
  Bin/1 -> Data Store Write1/1
  Data Store Read1/1 -> Cout/1
  empty/1 -> Logical Operator/1
  Data Type Conversion/1 -> read_assert/1
  Logical Operator/1 -> Data Type Conversion/1

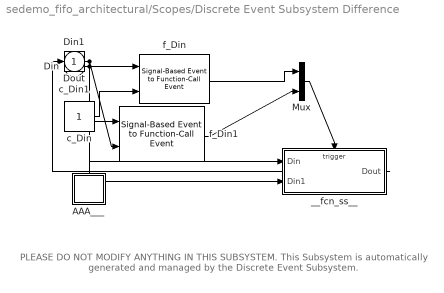
== system sedemo_fifo_architectural/Scopes/Discrete Event Subsystem Difference ==
  note: PLEASE DO NOT MODIFY ANYTHING IN THIS SUBSYSTEM.
      | This Subsystem is automatically generated and
      | managed by the Discrete Event Subsystem.
  Din : Inport  DataType=double  OutDataType=sfix(16)  OutScaling=2^0  OutDataTypeStr=double
  Din1 : Inport  Port=2  DataType=double  OutDataTypeStr=double
  AAA___ : Subsystem  LoadFcn=des_subsystemsupportblock(gcb, 'load');  InitFcn=des_subsystemsupportblock(gcb, 'init');  StartFcn=des_subsystemsupportblock(gcb, 'start');  StopFcn=des_subsystemsupportblock(gcb, 'stop');
      settings: CopyFcn=des_subsystemsupportblock(gcb, 'copy');  DeleteFcn=des_subsystemsupportblock(gcb, 'delete');  UndoDeleteFcn=des_subsystemsupportblock(gcb, 'undodelete');  ModelCloseFcn=des_subsystemsupportblock(gcb, 'modelclose');  PreSaveFcn=des_subsystemsupportblock(gcb, 'presave');  NameChangeFcn=des_subsystemsupportblock(gcb, 'namechange');  OpenFcn=des_subsystemsupportblock(gcb, 'open');  ParentCloseFcn=des_subsystemsupportblock(gcb, 'parentclose');
  Mux : Mux  Inputs=2
  __fcn_ss__ : Subsystem  TreatAsAtomicUnit=on
      settings: PropExecContextOutsideSubsystem=on
  c_Din : Constant  OutDataType=sfix(16)  OutScaling=2^0
  c_Din1 : Constant
  f_Din : simeventstranslate1/Signal-Based Event to Function-Call Event  Priority=1  SystemSampleTime=-1  GenerateFunctionCallUpon=Sample time hit from port ts  SignalEdgeOption=Rising  EnableE1Port=on  EnableF2Port=off  EnableE2Port=off  SpecifyEventPriority=off  PriorityFunctionCall=20  FunctionCallDelayFrom=Dialog  DelayFunctionCall=0  StatNumberF1Calls=Off  StatNumberF2Calls=Off  MaskBlockType=DESS_EVENT_PORT
  f_Din1 : simeventstranslate1/Signal-Based Event to Function-Call Event  Priority=1  SystemSampleTime=-1  GenerateFunctionCallUpon=Sample time hit from port ts  SignalEdgeOption=Rising  EnableE1Port=on  EnableF2Port=off  EnableE2Port=off  SpecifyEventPriority=off  PriorityFunctionCall=20  FunctionCallDelayFrom=Dialog  DelayFunctionCall=0  StatNumberF1Calls=Off  StatNumberF2Calls=Off  MaskBlockType=DESS_EVENT_PORT
  Dout : Outport
  wires:
  f_Din/1 -> Mux/1
  c_Din/1 -> f_Din/2
  Mux/1 -> __fcn_ss__/Trigger
  __fcn_ss__/1(Dout) -> Dout/1
  f_Din1/1 -> Mux/2
  c_Din1/1 -> f_Din1/2
  Din/1 -> f_Din/1, __fcn_ss__/1(Din)
  Din1/1 -> f_Din1/1, __fcn_ss__/2(Din1)

== system sedemo_fifo_architectural/FIFO Buffer/AND/AAA___ ==

== system sedemo_fifo_architectural/FIFO Buffer/AND/__fcn_ss__ ==
  Din : Inport  LoadFcn=des_subsysteminport(gcb, 'load');  InitFcn=des_subsysteminport(gcb, 'init');  StartFcn=des_subsysteminport(gcb, 'start');  StopFcn=des_subsysteminport(gcb, 'stop');  OutDataType=sfix(16)  OutScaling=2^0  mask(Discrete Event Inport){PermitSubsystemEvents=on, TypeOfEvent=Sample time hit, SignalEdgeOption=Rising, SpecifyEventPriority=off, PrioritySubsystemEvent=20}
      mask prompts: PermitSubsystemEvents "Execute subsystem upon signal-based events"; TypeOfEvent "Type of signal-based event:"; SignalEdgeOption "Type of change in signal value:"; SpecifyEventPriority "Resolve simultaneous signal updates according to event priority"; PrioritySubsystemEvent "Event priority:"
      mask help: Input port for a Discrete Event Subsystem block. This block can conditionally execute the subsystem upon signal-based events that meet specified criteria.
      mask init:
      | des_subsystemmask(gcb, 'init','apply')
      settings: CopyFcn=des_subsysteminport(gcb, 'copy');  DeleteFcn=des_subsysteminport(gcb, 'delete');  UndoDeleteFcn=des_subsysteminport(gcb, 'undodelete');  ModelCloseFcn=des_subsysteminport(gcb, 'modelclose');  PreSaveFcn=des_subsysteminport(gcb, 'presave');  NameChangeFcn=des_subsysteminport(gcb, 'namechange');  ParentCloseFcn=des_subsysteminport(gcb, 'parentclose');
      mask Help: helpview(simeventsbhelp);
      mask StyleString: checkbox,popup(Change in signal|Trigger|Sample time hit),popup(Rising|Falling|Either),checkbox,edit
      mask CallbackString: des_subsystemmask(gcb, 'cbPermitSubsystemEvents', 'noapply');|des_subsystemmask(gcb,'cbTypeOfEvent','noapply');||des_subsystemmask(gcb, 'cbSpecifyEventPriority', 'noapply');|
  Din1 : Inport  LoadFcn=des_subsysteminport(gcb, 'load');  InitFcn=des_subsysteminport(gcb, 'init');  StartFcn=des_subsysteminport(gcb, 'start');  StopFcn=des_subsysteminport(gcb, 'stop');  Port=2  OutDataType=sfix(16)  OutScaling=2^0  mask(Discrete Event Inport){PermitSubsystemEvents=on, TypeOfEvent=Sample time hit, SignalEdgeOption=Rising, SpecifyEventPriority=off, PrioritySubsystemEvent=20}
      mask prompts: PermitSubsystemEvents "Execute subsystem upon signal-based events"; TypeOfEvent "Type of signal-based event:"; SignalEdgeOption "Type of change in signal value:"; SpecifyEventPriority "Resolve simultaneous signal updates according to event priority"; PrioritySubsystemEvent "Event priority:"
      mask help: Input port for a Discrete Event Subsystem block. This block can conditionally execute the subsystem upon signal-based events that meet specified criteria.
      mask init:
      | des_subsystemmask(gcb, 'init','apply')
      settings: CopyFcn=des_subsysteminport(gcb, 'copy');  DeleteFcn=des_subsysteminport(gcb, 'delete');  UndoDeleteFcn=des_subsysteminport(gcb, 'undodelete');  ModelCloseFcn=des_subsysteminport(gcb, 'modelclose');  PreSaveFcn=des_subsysteminport(gcb, 'presave');  NameChangeFcn=des_subsysteminport(gcb, 'namechange');  ParentCloseFcn=des_subsysteminport(gcb, 'parentclose');
      mask Help: helpview(simeventsbhelp);
      mask StyleString: checkbox,popup(Change in signal|Trigger|Sample time hit),popup(Rising|Falling|Either),checkbox,edit
      mask CallbackString: des_subsystemmask(gcb, 'cbPermitSubsystemEvents', 'noapply');|des_subsystemmask(gcb,'cbTypeOfEvent','noapply');||des_subsystemmask(gcb, 'cbSpecifyEventPriority', 'noapply');|
  Subsystem Configuration : TriggerPort  TriggerType=function-call
      settings: CopyFcn=des_subsystemconfigblock(gcb, 'copy');  DeleteFcn=des_subsystemconfigblock(gcb, 'delete');  UndoDeleteFcn=des_subsystemconfigblock(gcb, 'undodelete');
      mask Type: Subsystem Configuration
      mask Description: Configuration for a Discrete Event Subsystem block. Every discrete event subsystem window must contain exactly one copy of this configuration block. Do not delete this block.
      mask Help: helpview(simeventsbhelp);
      mask Display: disp('Do Not Delete');
  Data Type Conversion2 : DataTypeConversion  OutDataType=sfix(16)  OutScaling=2^0
  Logical Operator1 : Logic  AllPortsSameDT=off  OutDataTypeMode=boolean  OutDataTypeStr=boolean
  Dout : Outport  LoadFcn=des_subsystemoutport(gcb, 'load');  InitFcn=des_subsystemoutport(gcb, 'init');  StartFcn=des_subsystemoutport(gcb, 'start');  StopFcn=des_subsystemoutport(gcb, 'stop');  OutDataType=sfix(16)  OutScaling=2^0
      settings: CopyFcn=des_subsystemoutport(gcb, 'copy');  DeleteFcn=des_subsystemoutport(gcb, 'delete');  UndoDeleteFcn=des_subsystemoutport(gcb, 'undodelete');  ModelCloseFcn=des_subsystemoutport(gcb, 'modelclose');  PreSaveFcn=des_subsystemoutport(gcb, 'presave');  NameChangeFcn=des_subsystemoutport(gcb, 'namechange');  ParentCloseFcn=des_subsystemoutport(gcb, 'parentclose');
      mask Type: Discrete Event Outport
      mask Description: Provide an output port for a Discrete Event Subsystem block.
      mask Help: helpview(simeventsbhelp);
  wires:
  Din/1 -> Logical Operator1/1
  Din1/1 -> Logical Operator1/2
  Logical Operator1/1 -> Data Type Conversion2/1
  Data Type Conversion2/1 -> Dout/1

== system sedemo_fifo_architectural/FIFO Buffer/AND1/AAA___ ==

== system sedemo_fifo_architectural/FIFO Buffer/AND1/__fcn_ss__ ==
  Din : Inport  LoadFcn=des_subsysteminport(gcb, 'load');  InitFcn=des_subsysteminport(gcb, 'init');  StartFcn=des_subsysteminport(gcb, 'start');  StopFcn=des_subsysteminport(gcb, 'stop');  OutDataType=sfix(16)  OutScaling=2^0  mask(Discrete Event Inport){PermitSubsystemEvents=on, TypeOfEvent=Sample time hit, SignalEdgeOption=Rising, SpecifyEventPriority=off, PrioritySubsystemEvent=20}
      mask prompts: PermitSubsystemEvents "Execute subsystem upon signal-based events"; TypeOfEvent "Type of signal-based event:"; SignalEdgeOption "Type of change in signal value:"; SpecifyEventPriority "Resolve simultaneous signal updates according to event priority"; PrioritySubsystemEvent "Event priority:"
      mask help: Input port for a Discrete Event Subsystem block. This block can conditionally execute the subsystem upon signal-based events that meet specified criteria.
      mask init:
      | des_subsystemmask(gcb, 'init','apply')
      settings: CopyFcn=des_subsysteminport(gcb, 'copy');  DeleteFcn=des_subsysteminport(gcb, 'delete');  UndoDeleteFcn=des_subsysteminport(gcb, 'undodelete');  ModelCloseFcn=des_subsysteminport(gcb, 'modelclose');  PreSaveFcn=des_subsysteminport(gcb, 'presave');  NameChangeFcn=des_subsysteminport(gcb, 'namechange');  ParentCloseFcn=des_subsysteminport(gcb, 'parentclose');
      mask Help: helpview(simeventsbhelp);
      mask StyleString: checkbox,popup(Change in signal|Trigger|Sample time hit),popup(Rising|Falling|Either),checkbox,edit
      mask CallbackString: des_subsystemmask(gcb, 'cbPermitSubsystemEvents', 'noapply');|des_subsystemmask(gcb,'cbTypeOfEvent','noapply');||des_subsystemmask(gcb, 'cbSpecifyEventPriority', 'noapply');|
  Din1 : Inport  LoadFcn=des_subsysteminport(gcb, 'load');  InitFcn=des_subsysteminport(gcb, 'init');  StartFcn=des_subsysteminport(gcb, 'start');  StopFcn=des_subsysteminport(gcb, 'stop');  Port=2  OutDataType=sfix(16)  OutScaling=2^0  mask(Discrete Event Inport){PermitSubsystemEvents=on, TypeOfEvent=Sample time hit, SignalEdgeOption=Rising, SpecifyEventPriority=off, PrioritySubsystemEvent=20}
      mask prompts: PermitSubsystemEvents "Execute subsystem upon signal-based events"; TypeOfEvent "Type of signal-based event:"; SignalEdgeOption "Type of change in signal value:"; SpecifyEventPriority "Resolve simultaneous signal updates according to event priority"; PrioritySubsystemEvent "Event priority:"
      mask help: Input port for a Discrete Event Subsystem block. This block can conditionally execute the subsystem upon signal-based events that meet specified criteria.
      mask init:
      | des_subsystemmask(gcb, 'init','apply')
      settings: CopyFcn=des_subsysteminport(gcb, 'copy');  DeleteFcn=des_subsysteminport(gcb, 'delete');  UndoDeleteFcn=des_subsysteminport(gcb, 'undodelete');  ModelCloseFcn=des_subsysteminport(gcb, 'modelclose');  PreSaveFcn=des_subsysteminport(gcb, 'presave');  NameChangeFcn=des_subsysteminport(gcb, 'namechange');  ParentCloseFcn=des_subsysteminport(gcb, 'parentclose');
      mask Help: helpview(simeventsbhelp);
      mask StyleString: checkbox,popup(Change in signal|Trigger|Sample time hit),popup(Rising|Falling|Either),checkbox,edit
      mask CallbackString: des_subsystemmask(gcb, 'cbPermitSubsystemEvents', 'noapply');|des_subsystemmask(gcb,'cbTypeOfEvent','noapply');||des_subsystemmask(gcb, 'cbSpecifyEventPriority', 'noapply');|
  Subsystem Configuration : TriggerPort  TriggerType=function-call
      settings: CopyFcn=des_subsystemconfigblock(gcb, 'copy');  DeleteFcn=des_subsystemconfigblock(gcb, 'delete');  UndoDeleteFcn=des_subsystemconfigblock(gcb, 'undodelete');
      mask Type: Subsystem Configuration
      mask Description: Configuration for a Discrete Event Subsystem block. Every discrete event subsystem window must contain exactly one copy of this configuration block. Do not delete this block.
      mask Help: helpview(simeventsbhelp);
      mask Display: disp('Do Not Delete');
  Data Type Conversion2 : DataTypeConversion  OutDataType=sfix(16)  OutScaling=2^0
  Logical Operator1 : Logic  AllPortsSameDT=off  OutDataTypeMode=boolean  OutDataTypeStr=boolean
  Dout : Outport  LoadFcn=des_subsystemoutport(gcb, 'load');  InitFcn=des_subsystemoutport(gcb, 'init');  StartFcn=des_subsystemoutport(gcb, 'start');  StopFcn=des_subsystemoutport(gcb, 'stop');  OutDataType=sfix(16)  OutScaling=2^0
      settings: CopyFcn=des_subsystemoutport(gcb, 'copy');  DeleteFcn=des_subsystemoutport(gcb, 'delete');  UndoDeleteFcn=des_subsystemoutport(gcb, 'undodelete');  ModelCloseFcn=des_subsystemoutport(gcb, 'modelclose');  PreSaveFcn=des_subsystemoutport(gcb, 'presave');  NameChangeFcn=des_subsystemoutport(gcb, 'namechange');  ParentCloseFcn=des_subsystemoutport(gcb, 'parentclose');
      mask Type: Discrete Event Outport
      mask Description: Provide an output port for a Discrete Event Subsystem block.
      mask Help: helpview(simeventsbhelp);
  wires:
  Din/1 -> Logical Operator1/1
  Din1/1 -> Logical Operator1/2
  Logical Operator1/1 -> Data Type Conversion2/1
  Data Type Conversion2/1 -> Dout/1

== system sedemo_fifo_architectural/FIFO Buffer/Compare to Thresholds/AAA___ ==
